simulink model "Lab3_Simulation_Wind"  (R2016a)
settings: Solver=VariableStepAuto  StartTime=0.0  StopTime=3  MaxStep=0.001  RelTol=1e-3
settings Model: Creator=Tomas  LastModifiedBy=Tomas

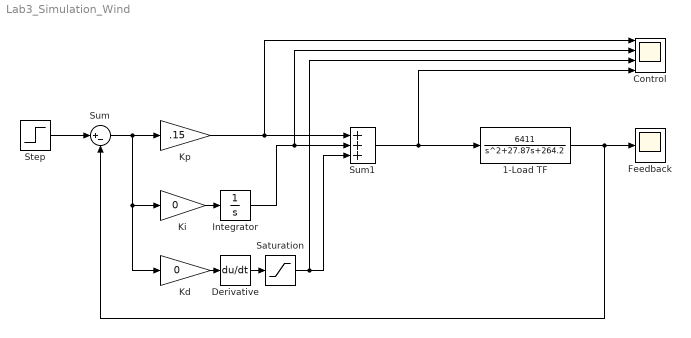
== system Lab3_Simulation_Wind ==
  1-Load TF : TransferFcn  Numerator=[6411]  Denominator=[1 27.87 264.2]
  Control : Scope  NumInputPorts=4
  Derivative : Derivative
  Feedback : Scope
  Integrator : Integrator
  Kd : Gain  Gain=0
  Ki : Gain  Gain=0
  Kp : Gain  Gain=.15
  Saturation : Saturate  UpperLimit=12  LowerLimit=-12
  Step : Step  After=45  SampleTime=0
  Sum : Sum  Inputs=|+-
  Sum1 : Sum  Inputs=+++
  wires:
  Step/1 -> Sum/1
  Sum/1 -> Kd/1, Ki/1, Kp/1
  Ki/1 -> Integrator/1
  Kp/1 -> Control/1, Sum1/1
  Integrator/1 -> Control/2, Sum1/2
  1-Load TF/1 -> Feedback/1, Sum/2
  Kd/1 -> Derivative/1
  Sum1/1 -> Control/4, 1-Load TF/1
  Derivative/1 -> Saturation/1
  Saturation/1 -> Control/3, Sum1/3
